simulink model "Overtaking"  (R2024a)
settings: Solver=FixedStepDiscrete  StartTime=0.0  StopTime=inf  FixedStep=0.001  RelTol=1e-3  EnableMultiTasking=on
undefined symbols (not defined in the file): route1_frenet, route1_waypoint, route2_frenet, route2_waypoint, route3_frenet, route3_waypoint, route4_frenet, route4_waypoint, route5_frenet, route5_waypoint
libraries: CarMaker4SL x46, simulink x1, slpidlib x1
(part 3 of 3)

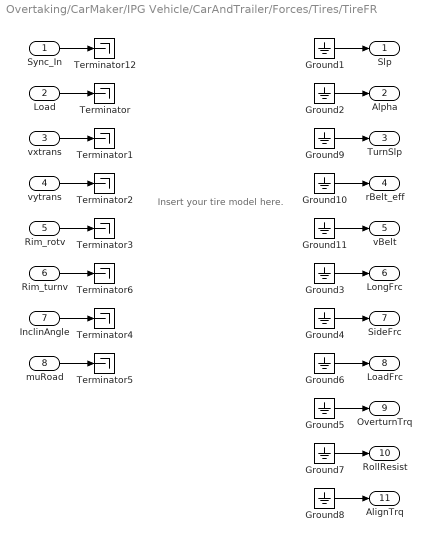
== system Overtaking/CarMaker/IPG Vehicle/CarAndTrailer/Forces/Tires/TireFR ==
  note: Insert your tire model here.
  Sync_In : Inport
  Load : Inport  Port=2
  vxtrans : Inport  Port=3
  vytrans : Inport  Port=4
  Rim_rotv : Inport  Port=5
  Rim_turnv : Inport  Port=6
  InclinAngle : Inport  Port=7
  muRoad : Inport  Port=8
  Ground{1..11} (11 alike) : Ground
  Terminator{,1..6,12} (8 alike) : Terminator
  Slp : Outport  VectorParamsAs1DForOutWhenUnconnected=off
  Alpha : Outport  Port=2  VectorParamsAs1DForOutWhenUnconnected=off
  TurnSlp : Outport  Port=3  VectorParamsAs1DForOutWhenUnconnected=off
  rBelt_eff : Outport  Port=4  VectorParamsAs1DForOutWhenUnconnected=off
  vBelt : Outport  Port=5  VectorParamsAs1DForOutWhenUnconnected=off
  LongFrc : Outport  Port=6  VectorParamsAs1DForOutWhenUnconnected=off
  SideFrc : Outport  Port=7  VectorParamsAs1DForOutWhenUnconnected=off
  LoadFrc : Outport  Port=8  VectorParamsAs1DForOutWhenUnconnected=off
  OverturnTrq : Outport  Port=9  VectorParamsAs1DForOutWhenUnconnected=off
  RollResist : Outport  Port=10  VectorParamsAs1DForOutWhenUnconnected=off
  AlignTrq : Outport  Port=11  VectorParamsAs1DForOutWhenUnconnected=off
  wires:
  Ground11/1 -> vBelt/1
  Ground10/1 -> rBelt_eff/1
  Ground9/1 -> TurnSlp/1
  Rim_turnv/1 -> Terminator6/1
  Sync_In/1 -> Terminator12/1
  Ground2/1 -> Alpha/1
  Ground3/1 -> LongFrc/1
  Ground4/1 -> SideFrc/1
  Ground5/1 -> OverturnTrq/1
  vxtrans/1 -> Terminator1/1
  vytrans/1 -> Terminator2/1
  Rim_rotv/1 -> Terminator3/1
  InclinAngle/1 -> Terminator4/1
  muRoad/1 -> Terminator5/1
  Load/1 -> Terminator/1
  Ground1/1 -> Slp/1
  Ground6/1 -> LoadFrc/1
  Ground7/1 -> RollResist/1
  Ground8/1 -> AlignTrq/1

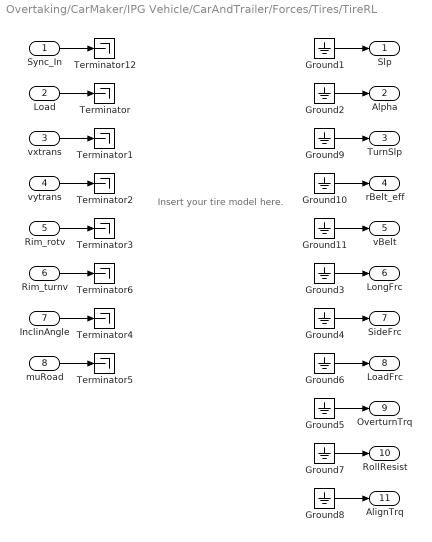
== system Overtaking/CarMaker/IPG Vehicle/CarAndTrailer/Forces/Tires/TireRL ==
  note: Insert your tire model here.
  Sync_In : Inport
  Load : Inport  Port=2
  vxtrans : Inport  Port=3
  vytrans : Inport  Port=4
  Rim_rotv : Inport  Port=5
  Rim_turnv : Inport  Port=6
  InclinAngle : Inport  Port=7
  muRoad : Inport  Port=8
  Ground{1..11} (11 alike) : Ground
  Terminator{,1..6,12} (8 alike) : Terminator
  Slp : Outport  VectorParamsAs1DForOutWhenUnconnected=off
  Alpha : Outport  Port=2  VectorParamsAs1DForOutWhenUnconnected=off
  TurnSlp : Outport  Port=3  VectorParamsAs1DForOutWhenUnconnected=off
  rBelt_eff : Outport  Port=4  VectorParamsAs1DForOutWhenUnconnected=off
  vBelt : Outport  Port=5  VectorParamsAs1DForOutWhenUnconnected=off
  LongFrc : Outport  Port=6  VectorParamsAs1DForOutWhenUnconnected=off
  SideFrc : Outport  Port=7  VectorParamsAs1DForOutWhenUnconnected=off
  LoadFrc : Outport  Port=8  VectorParamsAs1DForOutWhenUnconnected=off
  OverturnTrq : Outport  Port=9  VectorParamsAs1DForOutWhenUnconnected=off
  RollResist : Outport  Port=10  VectorParamsAs1DForOutWhenUnconnected=off
  AlignTrq : Outport  Port=11  VectorParamsAs1DForOutWhenUnconnected=off
  wires:
  Ground11/1 -> vBelt/1
  Ground10/1 -> rBelt_eff/1
  Ground9/1 -> TurnSlp/1
  Rim_turnv/1 -> Terminator6/1
  Sync_In/1 -> Terminator12/1
  Ground2/1 -> Alpha/1
  Ground3/1 -> LongFrc/1
  Ground4/1 -> SideFrc/1
  Ground5/1 -> OverturnTrq/1
  vxtrans/1 -> Terminator1/1
  vytrans/1 -> Terminator2/1
  Rim_rotv/1 -> Terminator3/1
  InclinAngle/1 -> Terminator4/1
  muRoad/1 -> Terminator5/1
  Load/1 -> Terminator/1
  Ground1/1 -> Slp/1
  Ground6/1 -> LoadFrc/1
  Ground7/1 -> RollResist/1
  Ground8/1 -> AlignTrq/1

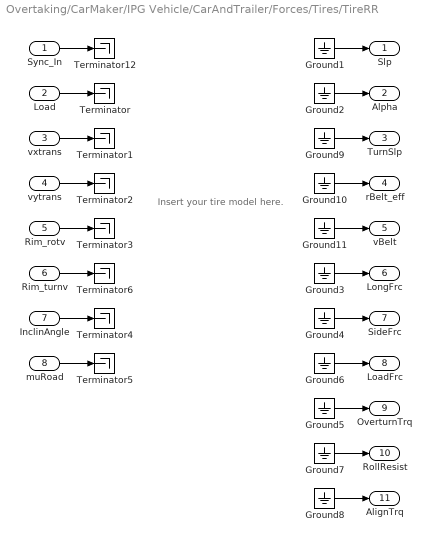
== system Overtaking/CarMaker/IPG Vehicle/CarAndTrailer/Forces/Tires/TireRR ==
  note: Insert your tire model here.
  Sync_In : Inport
  Load : Inport  Port=2
  vxtrans : Inport  Port=3
  vytrans : Inport  Port=4
  Rim_rotv : Inport  Port=5
  Rim_turnv : Inport  Port=6
  InclinAngle : Inport  Port=7
  muRoad : Inport  Port=8
  Ground{1..11} (11 alike) : Ground
  Terminator{,1..6,12} (8 alike) : Terminator
  Slp : Outport  VectorParamsAs1DForOutWhenUnconnected=off
  Alpha : Outport  Port=2  VectorParamsAs1DForOutWhenUnconnected=off
  TurnSlp : Outport  Port=3  VectorParamsAs1DForOutWhenUnconnected=off
  rBelt_eff : Outport  Port=4  VectorParamsAs1DForOutWhenUnconnected=off
  vBelt : Outport  Port=5  VectorParamsAs1DForOutWhenUnconnected=off
  LongFrc : Outport  Port=6  VectorParamsAs1DForOutWhenUnconnected=off
  SideFrc : Outport  Port=7  VectorParamsAs1DForOutWhenUnconnected=off
  LoadFrc : Outport  Port=8  VectorParamsAs1DForOutWhenUnconnected=off
  OverturnTrq : Outport  Port=9  VectorParamsAs1DForOutWhenUnconnected=off
  RollResist : Outport  Port=10  VectorParamsAs1DForOutWhenUnconnected=off
  AlignTrq : Outport  Port=11  VectorParamsAs1DForOutWhenUnconnected=off
  wires:
  Ground11/1 -> vBelt/1
  Ground10/1 -> rBelt_eff/1
  Ground9/1 -> TurnSlp/1
  Rim_turnv/1 -> Terminator6/1
  Sync_In/1 -> Terminator12/1
  Ground2/1 -> Alpha/1
  Ground3/1 -> LongFrc/1
  Ground4/1 -> SideFrc/1
  Ground5/1 -> OverturnTrq/1
  vxtrans/1 -> Terminator1/1
  vytrans/1 -> Terminator2/1
  Rim_rotv/1 -> Terminator3/1
  InclinAngle/1 -> Terminator4/1
  muRoad/1 -> Terminator5/1
  Load/1 -> Terminator/1
  Ground1/1 -> Slp/1
  Ground6/1 -> LoadFrc/1
  Ground7/1 -> RollResist/1
  Ground8/1 -> AlignTrq/1

== matlab function Overtaking/CarMaker/Subsystem/Final Project/Scenario 1/MATLAB Function5 ==
  data: route input; candidate_paths output; route1_frenet input; route3_frenet input; ego_s input; ego_d input
function candidate_paths = generate_candidate_paths(route, route1_frenet, route3_frenet, ego_s, ego_d)
    global_s = route(:,1);
    global_d = route(:,2);
    
    % lane_width를 고정값으로 가정
    lane_width = 6;
    num_lateral_paths = 9;  % 반드시 홀수 (중앙값이 0이 되도록)
    
    % d
    % 왼쪽이 양수
    % 오른쪽이 음수
    
    % 중앙값이 0이 되도록 등간격 리스트 생성
    half_range = lane_width/2;
    step = 2 * half_range / (num_lateral_paths - 1);
    deviation_list = -half_range : step : half_range;
    
    if isequal(route, route1_frenet)
        if ego_d > 0
            deviation_list(deviation_list > 0) = 0; % 차량이 왼쪽 차선의 바깥쪽에 붙은 경우 중앙~오른쪽만 허용
        end 
    end
    
    if isequal(route, route3_frenet)
        if ego_d < 0
            deviation_list(deviation_list < 0) = 0;  % 차량이 오른쪽 차선의 바깥쪽에 붙은 경우 차선은 중앙~왼쪽만 허용
        end
    end
    
    % 경로 설정 파라미터
    lookahead_index  = 5;          % lookahead_index
    num_points = 20;
    
    candidate_paths = generate_candidate_paths_func( ...
        global_s, global_d, ego_s, ego_d, deviation_list, lookahead_index , num_points);
end

== matlab function Overtaking/CarMaker/Subsystem/Final Project/Scenario 1/MATLAB Function7 ==
  data: candidate_paths input; path_costs output; opt_d input; target_speed input; dt input; s_path output; d_path output
function [path_costs, s_path, d_path] = calculate_path_costs(candidate_paths, opt_d, target_speed, dt)

    path_costs = calculate_path_costs_func(candidate_paths, opt_d, target_speed, dt);    % 후보 경로마다 cost 계산
    [s_path, d_path] = select_lowest_cost_path(candidate_paths, path_costs);        % minimum cost인 경로 (s, d) 추출
    
    % d_path_len : 20
    % s_path_len : 20
end

== matlab function Overtaking/CarMaker/Subsystem/Final Project/Scenario 1/MATLAB Function8 ==
  data: optimal_path input; cartesian_path output; route_waypoints input; num_points output
function [cartesian_path, num_points] = convert_all_frenet_to_cartesian(optimal_path, route_waypoints)

    [cartesian_path, num_points] = convert_all_frenet_to_cartesian_func(optimal_path, route_waypoints);
end

== matlab function Overtaking/CarMaker/Subsystem/Final Project/Scenario 1/MATLAB Function6 ==
  data: valid_idx input; optimal_path output; candidates_cost input; candidate_paths_cartesian input; num_points output; best_idx output; candidates_cost output
function [optimal_path, num_points, best_idx, candidates_cost] = collision_check(valid_idx, candidates_cost, candidate_paths_cartesian)

    [optimal_path, num_points, best_idx, candidates_cost] = collision_check_func(valid_idx, candidates_cost, candidate_paths_cartesian);
end

== matlab function Overtaking/CarMaker/Subsystem/Final Project/Scenario 1/Subsystem3/MATLAB Function ==
  data: waypoints input; local_waypoints_ output; vehicle_position input; head input; path_len input
function local_waypoints_ = global_to_local_waypoints(waypoints, vehicle_position, head, path_len)
    % 로컬 좌표 변환 함수 (yaw 변화가 작으면 무시)
    % 입력:
    %   waypoints        : [N x 2] 전체 전역 경로
    %   vehicle_position : [1 x 2] 자차 위치 [x, y]
    %   head             : 자차 yaw [rad]
    %   path_len         : 유효 경로 길이

    local_waypoints_ = zeros(400, 2);  % Simulink 고정 크기 호환

 

    x_ego = vehicle_position(1);
    y_ego = vehicle_position(2);

    waypoints_x = waypoints(:, 1);
    waypoints_y = waypoints(:, 2);

    % --- 전체 경로를 로컬 좌표계로 변환 ---
    for i = 1:path_len
        dx = waypoints_x(i) - x_ego;
        dy = waypoints_y(i) - y_ego;

        x_local = dx * cos(-head) - dy * sin(-head);
        y_local = dx * sin(-head) + dy * cos(-head);

        local_waypoints_(i, :) = [x_local, y_local];
    end
end

== matlab function Overtaking/CarMaker/Subsystem/Final Project/Scenario 1/Subsystem3/MATLAB Function2 ==
  data: poly_coeff input; target_velocity output; lookahead input
function target_velocity = longitudinal_speed_control_from_poly(poly_coeff, lookahead)
    V_max = 30.0/3.6;
    % V_max = 50.0/3.6;
    
    x_for_curv = lookahead;

    % 곡률 계산
    dy_dx   = polyval(polyder(poly_coeff), x_for_curv);
    d2y_dx2 = polyval(polyder(polyder(poly_coeff)), x_for_curv);
    kappa = d2y_dx2 / (1 + dy_dx^2)^(3/2);



    v_from_curvature = V_max * exp(-5.0 * abs(kappa));
    v = v_from_curvature;


    target_velocity = v;

    % % ======== 저역통과 필터 (optional) =========
    % persistent prev_v
    % if isempty(prev_v)
    %     prev_v = v;
    % end
    % 
    % alpha = 0.95;  % 0.85~0.95 추천 (1에 가까울수록 부드럽고 느림)
    % target_velocity = alpha * prev_v + (1 - alpha) * v;
    % prev_v = target_velocity;
end

== matlab function Overtaking/CarMaker/Subsystem/Final Project/Scenario 1/Subsystem3/MATLAB Function3 ==
  data: poly_coeff input; steering_angle output; velocity input; x_lookahead output
function [steering_angle, x_lookahead] = adaptive_pure_pursuit_from_poly(poly_coeff, velocity)
% Adaptive Pure Pursuit with dynamic lookahead based on velocity and curvature
% 입력:
%   poly_coeff : 경로 다항식 계수 [1x4] (y = ax^3 + bx^2 + cx + d)
%   velocity   : 자차 속도 [m/s]
% 출력:
%   steering_angle : 조향각 [rad]
%   x_lookahead    : lookahead 거리 [m]

    % 차량 파라미터
    L = 2.9;  % 차량 휠베이스 [m]

    % Lookahead 계산 파라미터
    Lxd = 2.5;       % 기본 lookahead [m]
    kv = 0.8;        % 속도 계수
    kc = 1;       % 곡률 보정 계수
    rad2deg = 180 / pi;

    % 곡률 평가 위치 (예: x=3.0)에서 곡률 추정
    x_for_curv = 3.0;
    dy_dx  = polyval(polyder(poly_coeff), x_for_curv);
    d2y_dx2 = polyval(polyder(polyder(poly_coeff)), x_for_curv);
    curvature = d2y_dx2 / (1 + dy_dx^2)^(3/2);  % 곡률

    % lookahead 거리 계산
    x_lookahead = Lxd + kv * velocity - kc * abs(curvature * rad2deg);
    x_lookahead = max(2.0, x_lookahead);  % 최소 거리 제한

    % lookahead 위치에서 목표점 좌표
    y_target = polyval(poly_coeff, x_lookahead);

    % 좌표 기반 조향각 계산 (Pure Pursuit 방식)
    alpha = atan2(y_target, x_lookahead);  % heading error
    steering_angle = atan2(2 * L * sin(alpha), x_lookahead);


    
end

== matlab function Overtaking/CarMaker/Subsystem/Final Project/Scenario 1/Subsystem3/MATLAB Function1 ==
  data: local_waypoints input; poly_coeff output
function poly_coeff = fit_polynomial_to_waypoints(local_waypoints)
% 전방 포인트(x > 0) 중 y값 차이가 10 이하이며, y값이 -30~30 사이인 포인트만 사용

    % 1차 필터링: x > 0
    valid_idx = local_waypoints(:,1) > 0;
    filtered = local_waypoints(valid_idx, :);

    % 2차 필터링: y in [-8, 8]
    y_range_idx = abs(filtered(:,2)) <= 8;
    filtered = filtered(y_range_idx, :);

    % 앞쪽 30개만 사용
    N = min(5, size(filtered, 1));
    x = filtered(1:N, 1);
    y = filtered(1:N, 2);

    % 최소 포인트 수 확인 후 3차 다항식 피팅
    if length(x) >= 4
        poly_coeff = polyfit(x, y, 3);
    else
        poly_coeff = zeros(1, 4);
    end
end

== matlab function Overtaking/CarMaker/Subsystem/Final Project/Scenario 1/MATLAB Function10 ==
  data: traffic_info input; obs_xy output
function obs_xy = mux_traffics_xy(traffic_info)

    obs_xy = mux_traffics_xy_func(traffic_info);
end

== matlab function Overtaking/CarMaker/Subsystem/Final Project/Scenario 1/MATLAB Function ==
  data: waypoints input; EgoFrenet output; interval input; egoState input
function EgoFrenet = convertPathToFrenet(waypoints, interval, egoState)

    EgoFrenet = convertPathToFrenet(waypoints, interval, egoState);
end

== stateflow chart Overtaking/CarMaker/Subsystem/Day3/Chart ==
  (default) -> (junction 1)
  (junction 1) -> (junction 3) [order 1] : [i<99]
      | {i = i + 1;}
  (junction 1) -> (junction 7) [order 2] : {i=0;}
  (junction 3) -> (junction 5)
  (junction 5) -> (junction 7)
  (junction 7) -> (junction 10)
  (junction 10) -> (junction 12) [order 1] : [rem(i,50) == 0]
      | {do_Logic;}
  (junction 10) -> (junction 18) [order 2]
  (junction 12) -> (junction 16)
  (junction 16) -> (junction 18)
  (junction 18) -> (junction 21)
  data: i local =0
  events: do_Logic output FUNCTION_CALL_EVENT

== matlab function Overtaking/CarMaker/Subsystem/Final Project/Scenario 1/MATLAB Function1 ==
  data: lane_id input; route_waypoint output; route_frenet output; route1_waypoint input; route1_frenet input; route2_waypoint input; route2_frenet input; route3_waypoint input; route3_frenet input; route4_waypoint input; route4_frenet input; route5_waypoint input; route5_frenet input
function [route_waypoint, route_frenet] = select_lane(lane_id, route1_waypoint, ...
    route1_frenet, route2_waypoint, route2_frenet, route3_waypoint, route3_frenet, ...
    route4_waypoint, route4_frenet, route5_waypoint, route5_frenet)

    [route_waypoint, route_frenet] = select_lane_func(lane_id, route1_waypoint, ...
    route1_frenet, route2_waypoint, route2_frenet, route3_waypoint, route3_frenet, ...
    route4_waypoint, route4_frenet, route5_waypoint, route5_frenet);
end

== matlab function Overtaking/CarMaker/Subsystem/Final Project/Scenario 1/MATLAB Function2 ==
  data: candidate_paths_cartesian input; valid_idx output; obs_xy input
function valid_idx= apply_constraint_to_candidate(candidate_paths_cartesian, obs_xy)

    valid_idx = apply_constraint_to_candidate_func(candidate_paths_cartesian, obs_xy);

    % for i = 1:length(valid_idx)
    %     idx = valid_idx(i);
    %     valid_paths = candidate_paths_cartesian(:, :, idx);  % [N x 2] 크기
    % end
end

== matlab function Overtaking/CarMaker/Subsystem/Final Project/Scenario 1/MATLAB Function4 ==
  data: u input; Ego_s output; Ego_ds output; Ego_dds output; Ego_d output; Ego_dd output; Ego_ddd output
function [Ego_s, Ego_ds, Ego_dds, Ego_d, Ego_dd, Ego_ddd] = fcn(u)
    
    Ego_s = u(1);
    Ego_ds = u(2);
    Ego_dds = u(3);
    Ego_d = u(4);
    Ego_dd = u(5);
    Ego_ddd = u(6);

end
